simulink model "Simulink_asserv_Disc_15Mars"  (R2024a)
settings: Solver=VariableStepAuto  StartTime=0.0  StopTime=1000  FixedStep=0.01  RelTol=1e-3
model workspace (MAT data in the model file):
  AmbiantTemp = 25
  CondSig_mesureTemp_Gain = 4.35
  CondSig_mesureTemp_Vsub = 1.95
  DivTen_mesureTemp_R_pullup = 10000
  DivTen_mesureTemp_Vcc = 5
  Estimateur_alpha = 0.5
  Filtre_mesureTemp_deno = [0.0033 1]
  Gain_Comparateur_VoltageControle = 0.32
  RC_deno = [3.22e-08 3.04e-05 0.00955 1]
  SourceCourant_Gain_Vcontrole_vers_A = 3.1564
  ThermoRes_SHTEMP_A = 0.003354
  ThermoRes_SHTEMP_B = 0.00026
  ThermoRes_SHTEMP_C = 1.6e-06
  ThermoRes_SHTEMP_D = 6.3e-08
  ThermoRes_SH_A = -14.65719
  ThermoRes_SH_B = 4798.842
  ThermoRes_SH_C = -115334
  ThermoRes_SH_D = -3730535
  ThermoRes_SH_R_nom = 10000
  periodeEchant = 2
  setupDelay = 4
libraries: simulink x5
settings Model: SimulationMode=rapid-accelerator  Creator=alcot161  LastModifiedBy=ALCOT161

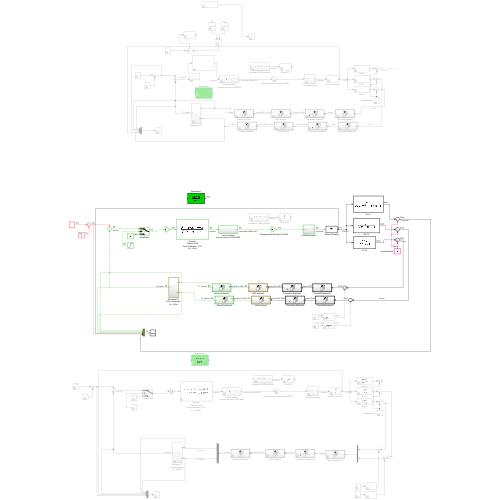
[thumbnail: Simulink's stored preview of the top-level diagram]
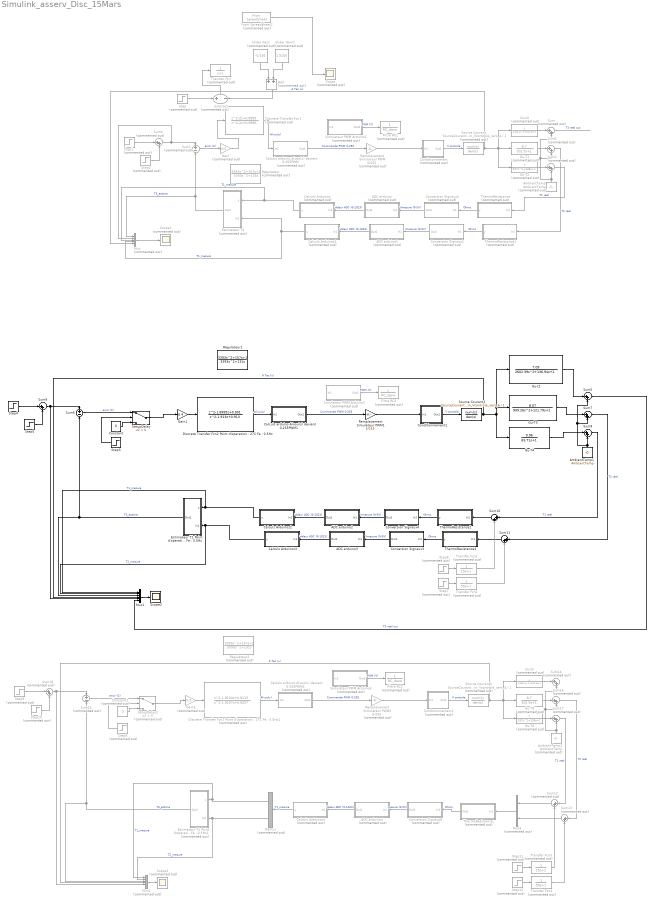
== system Simulink_asserv_Disc_15Mars ==
  ADC arduino : Subsystem  Commented=on  TreatAsAtomicUnit=on
  ADC arduino1 : Subsystem  Commented=on  TreatAsAtomicUnit=on
  ADC arduino2 : Subsystem  TreatAsAtomicUnit=on
  ADC arduino3 : Subsystem  TreatAsAtomicUnit=on
  ADC arduino4 : Subsystem  Commented=on  TreatAsAtomicUnit=on
  Add : Sum  Commented=on
  AmbiantTemp : Constant  Commented=on  Value=AmbiantTemp
  AmbiantTemp1 : Constant  Value=AmbiantTemp
  AmbiantTemp2 : Constant  Commented=on  Value=AmbiantTemp
  Calculs Arduinos : Subsystem  Commented=on  TreatAsAtomicUnit=on
  Calculs Arduinos1 : Subsystem  Commented=on  TreatAsAtomicUnit=on
  Calculs Arduinos2 : Subsystem  TreatAsAtomicUnit=on
  Calculs Arduinos3 : Subsystem  TreatAsAtomicUnit=on
  Calculs Arduinos4 : Subsystem  Commented=on  TreatAsAtomicUnit=on
  Calculs arduino A(voulu) devient 0-255PWM : Subsystem  Commented=on
  Calculs arduino A(voulu) devient 0-255PWM1 : Subsystem
  Calculs arduino A(voulu) devient 0-255PWM2 : Subsystem  Commented=on
  Conditionnement : Subsystem  Commented=on
  Conditionnement1 : Subsystem
  Conditionnement2 : Subsystem  Commented=on
  Constant : Constant  Value=0  SampleTime=periodeEchant
  Constant1 : Constant  Commented=on  Value=0  SampleTime=periodeEchant
  Conversion Signaux1 : Subsystem  Commented=on  TreatAsAtomicUnit=on
  Conversion Signaux2 : Subsystem  Commented=on  TreatAsAtomicUnit=on
  Conversion Signaux3 : Subsystem  TreatAsAtomicUnit=on
  Conversion Signaux4 : Subsystem  TreatAsAtomicUnit=on
  Conversion Signaux6 : Subsystem  Commented=on  TreatAsAtomicUnit=on
  Demux : Demux  Commented=on  Outputs=2
  Discrete Transfer Fcn1 : DiscreteTransferFcn  Commented=on  Numerator=[1 -2 0.9995]  Denominator=[1 -2 0.9996]
  "Discrete Transfer Fcn2 Point d'operation : 27C Fe : 0.5Hz" : DiscreteTransferFcn  Numerator=[1 -1.8995 0.901]  Denominator=[1 -1.913 0.913]
  "Discrete Transfer Fcn2 Point d'operation : 27C Fe : 0.5Hz1" : DiscreteTransferFcn  Commented=on  Numerator=[1 -1.9104 0.9115]  Denominator=[1 -1.9257 0.9257]
  "Estimateur T1 Point d'operation Fe : 0.5Hz" : Subsystem
  "Estimateur T1 Point d'operation Fe : 0.5Hz1" : Subsystem  Commented=on
  Estimateur T3 : Subsystem  Commented=on
  Filtre RC1 : TransferFcn  Commented=on  Denominator=RC_deno
  Filtre RC2 : TransferFcn  Commented=on  Denominator=RC_deno
  Filtre RC3 : TransferFcn  Commented=on  Denominator=RC_deno
  From Spreadsheet2 : FromSpreadsheet  Commented=on  FileName=N600_N800.xlsx  SheetName=P600_P800  Range=A2:A100  SampleTime=-1
  Gain : Gain  Commented=on  Gain=0.5
  Gain1 : Gain  Gain=0.4
  Gain2 : Gain  Commented=on  Gain=0.5
  Gu-T1 : TransferFcn  Commented=on  Numerator=[8.7]  Denominator=[102.5 1]
  Gu-T2 : TransferFcn  Commented=on  Numerator=[7]  Denominator=[537 138 1]
  Gu-T3 : TransferFcn  Numerator=[8.07]  Denominator=[909.26 121.79 1]
  Gu-T4 : TransferFcn  Numerator=[9.96]  Denominator=[83.71 1]
  Gu-T5 : TransferFcn  Commented=on  Numerator=[8.7]  Denominator=[102.5 1]
  Gu-T6 : TransferFcn  Commented=on  Numerator=[7]  Denominator=[537 138 1]
  Gu-t1 : TransferFcn  Numerator=[7.09]  Denominator=[2602.39 136.94 1]
  Gu-t2 : TransferFcn  Commented=on  Numerator=[6]  Denominator=[3403.4 156.9 1]
  Gu-t3 : TransferFcn  Commented=on  Numerator=[6]  Denominator=[3403.4 156.9 1]
  Mux : Mux  Commented=on  Inputs=5
  Mux1 : Mux  Inputs=6
  Mux2 : Mux  Commented=on  Inputs=6
  Mux3 : Mux  Commented=on  Inputs=2
  Remplacement Simulateur PWM : Gain  Commented=on  Gain=5/255
  Remplacement Simulateur PWM1 : Gain  Gain=5/255
  Remplacement Simulateur PWM2 : Gain  Commented=on  Gain=5/255
  Régulateur : TransferFcn  Commented=on  Numerator=[3393 157 1]  Denominator=[3393 131 0]
  Régulateur1 : TransferFcn  Numerator=[3393 157 1]  Denominator=[3393 131 0]
  Régulateur2 : TransferFcn  Commented=on  Numerator=[3393 157 1]  Denominator=[3393 131 0]
  Scope : Scope  Commented=on
  Scope1 : Scope  Commented=on
  Scope2 : Scope
  Scope3 : Scope  Commented=on
  SetupDelay : Switch  Criteria=u2 > Threshold  SaturateOnIntegerOverflow=off  InputSameDT=off
  SetupDelay1 : Switch  Commented=on  Criteria=u2 > Threshold  SaturateOnIntegerOverflow=off  InputSameDT=off
  Simulateur PWM Arduino1 : Subsystem  Commented=on
  Simulateur PWM Arduino2 : Subsystem  Commented=on
  Simulateur PWM Arduino3 : Subsystem  Commented=on
  Slider Gain : simulink/Math Operations/Slider Gain  Commented=on  gain=-0.516  low=-2  high=2
  Slider Gain1 : simulink/Math Operations/Slider Gain  Commented=on  gain=1.5155  low=-2  high=2
  Source Courant : TransferFcn  Commented=on  Numerator=SourceCourant_Gain_Vcontrole_vers_A  Denominator=1
  Source Courant1 : TransferFcn  Numerator=SourceCourant_Gain_Vcontrole_vers_A  Denominator=1
  Source Courant2 : TransferFcn  Commented=on  Numerator=SourceCourant_Gain_Vcontrole_vers_A  Denominator=1
  Step : Step  Commented=on  SampleTime=0
  Step1 : Step  Commented=on  Time=10  Before=25  After=27  SampleTime=0.05
  Step10 : Step  Commented=on  Time=500  After=-4  SampleTime=0.05
  Step11 : Step  Commented=on  Time=300  SampleTime=0
  Step12 : Step  Commented=on  Time=700  SampleTime=0
  Step2 : Step  Commented=on  Time=500  After=-4  SampleTime=0.05
  Step3 : Step  Time=setupDelay+1  SampleTime=periodeEchant
  Step4 : Step  Time=25  Before=25  After=27  SampleTime=0.05
  Step5 : Step  Time=500  After=-4  SampleTime=0.05
  Step6 : Step  Commented=on  Time=300  SampleTime=0
  Step7 : Step  Commented=on  Time=700  SampleTime=0
  Step8 : Step  Commented=on  Time=setupDelay+1  SampleTime=periodeEchant
  Step9 : Step  Commented=on  Time=25  Before=25  After=27  SampleTime=0.05
  Subtract : Sum  Commented=on  Inputs=+-
  Sum{,2..4,12..14,16..18} (10 alike) : Sum  Commented=on  Inputs=|++
  Sum1 : Sum  Commented=on  Inputs=+|-  SampleTime=0
  Sum{5,7..11} (6 alike) : Sum  Inputs=|++
  Sum15 : Sum  Commented=on  Inputs=+|-  SampleTime=2
  Sum6 : Sum  Inputs=+|-  SampleTime=2
  ThermoResistance : Subsystem  Commented=on  TreatAsAtomicUnit=on
  ThermoResistance1 : Subsystem  Commented=on  TreatAsAtomicUnit=on
  ThermoResistance2 : Subsystem  TreatAsAtomicUnit=on
  ThermoResistance3 : Subsystem  TreatAsAtomicUnit=on
  ThermoResistance_ : Subsystem  Commented=on  TreatAsAtomicUnit=on
  Transfer Fcn : TransferFcn  Commented=on  Denominator=[1 1]
  Transfer Fcn1 : TransferFcn  Commented=on  Denominator=[15 1]
  Transfer Fcn2 : TransferFcn  Commented=on  Denominator=[50 1]
  Transfer Fcn3 : TransferFcn  Commented=on  Denominator=[15 1]
  Transfer Fcn4 : TransferFcn  Commented=on  Denominator=[50 1]
  wires:
  From Spreadsheet2/1 -> Scope/1
  Subtract/1 -> Transfer Fcn/1
  Slider Gain/1 -> Add/1
  Slider Gain1/1 -> Add/2
  Add/1 -> Subtract/2
  Step/1 -> Subtract/1
  Sum1/1 -> Gain/1  "error (C)"
  Calculs arduino A(voulu) devient 0-255PWM/1(Out1) -> Remplacement Simulateur PWM/1  "Commande PWM 0-255"
  Remplacement Simulateur PWM/1 -> Conditionnement/1(In1)
  Conditionnement/1(Out1) -> Source Courant/1  "V controle"
  Source Courant/1 -> Mux/5, Gu-T2/1, Gu-T1/1, Gu-t3/1  "A Tec (u)"
  Gu-t3/1 -> Sum/1
  Gu-T1/1 -> Sum2/1
  Gu-T2/1 -> Sum3/1
  AmbiantTemp/1 -> Sum/2, Sum2/2, Sum3/2
  Sum2/1 -> ThermoResistance1/1(In1)  "T2 reel"
  Sum3/1 -> ThermoResistance/1(In1)  "T1 reel"
  ThermoResistance/1(y) -> Conversion Signaux2/1(In1)  "Ohms"
  Conversion Signaux2/1(Out1) -> ADC arduino/1(In1)  "Vmesure (0-5V)"
  ADC arduino/1(Out1) -> Calculs Arduinos/1(In1)  "Valeur ADC (0-1023)"
  Calculs Arduinos/1(y) -> Mux/3, Estimateur T3/1(y)  "T1_mesure"
  Estimateur T3/1(Out1) -> Mux/1, Sum1/2  "T3_estime"
  Simulateur PWM Arduino1/1(Out1) -> Filtre RC1/1  "PWM (V)"
  Sum/1 -> ?  "T3 reel out"
  Gain/1 -> Discrete Transfer Fcn1/1
  Discrete Transfer Fcn1/1 -> Calculs arduino A(voulu) devient 0-255PWM/1(In1)  "A(voulu)"
  Step1/1 -> Sum4/1
  Step2/1 -> Sum4/2
  Mux/1 -> Scope1/1
  Sum4/1 -> Mux/2, Sum1/1
  Calculs Arduinos1/1(y) -> Estimateur T3/2(In2), Mux/4  "T1_mesure"
  ThermoResistance1/1(y) -> Conversion Signaux1/1(In1)  "Ohms"
  ADC arduino1/1(Out1) -> Calculs Arduinos1/1(In1)  "Valeur ADC (0-1023)"
  Conversion Signaux1/1(Out1) -> ADC arduino1/1(In1)  "Vmesure (0-5V)"
  ThermoResistance3/1(y) -> Conversion Signaux3/1(In1)  "Ohms"
  Step4/1 -> Sum9/1
  Gu-T3/1 -> Sum7/1
  Conversion Signaux3/1(Out1) -> ADC arduino3/1(In1)  "Vmesure (0-5V)"
  Sum9/1 -> Sum6/1, Mux1/5
  ADC arduino3/1(Out1) -> Calculs Arduinos3/1(In1)  "Valeur ADC (0-1023)"
  Simulateur PWM Arduino2/1(Out1) -> Filtre RC2/1  "PWM (V)"
  Step5/1 -> Sum9/2
  Conversion Signaux4/1(Out1) -> ADC arduino2/1(In1)  "Vmesure (0-5V)"
  AmbiantTemp1/1 -> Sum5/2, Sum7/2, Sum8/2
  Remplacement Simulateur PWM1/1 -> Conditionnement1/1(In1)
  Calculs Arduinos2/1(y) -> Mux1/1, "Estimateur T1 Point d'operation Fe : 0.5Hz"/1(y)  "T1_mesure"
  ADC arduino2/1(Out1) -> Calculs Arduinos2/1(In1)  "Valeur ADC (0-1023)"
  Calculs arduino A(voulu) devient 0-255PWM1/1(Out1) -> Remplacement Simulateur PWM1/1  "Commande PWM 0-255"
  Calculs Arduinos3/1(y) -> Mux1/2, "Estimateur T1 Point d'operation Fe : 0.5Hz"/2(In2)  "T2_mesure"
  Source Courant1/1 -> Mux1/4, Gu-T3/1, Gu-t1/1, Gu-T4/1  "A Tec (u)"
  ThermoResistance2/1(y) -> Conversion Signaux4/1(In1)  "Ohms"
  Sum7/1 -> Sum11/1  "T2 reel"
  Conditionnement1/1(Out1) -> Source Courant1/1  "V controle"
  Gu-T4/1 -> Sum8/1
  Gu-t1/1 -> Sum5/1
  "Discrete Transfer Fcn2 Point d'operation : 27C Fe : 0.5Hz"/1 -> Calculs arduino A(voulu) devient 0-255PWM1/1(In1)  "A(voulu)"
  "Estimateur T1 Point d'operation Fe : 0.5Hz"/1(Out1) -> Mux1/3, Sum6/2  "T3_estime"
  Mux1/1 -> Scope2/1
  Step3/1 -> SetupDelay/2
  Gain1/1 -> "Discrete Transfer Fcn2 Point d'operation : 27C Fe : 0.5Hz"/1
  Sum6/1 -> SetupDelay/1  "error (C)"
  SetupDelay/1 -> Gain1/1
  Constant/1 -> SetupDelay/3
  Sum8/1 -> Sum10/1  "T1 reel"
  Step6/1 -> Transfer Fcn1/1
  Sum10/1 -> ThermoResistance2/1(In1)
  Sum11/1 -> ThermoResistance3/1(In1)
  Step7/1 -> Transfer Fcn2/1
  Transfer Fcn1/1 -> Sum10/2
  Transfer Fcn2/1 -> Sum11/2
  Transfer Fcn3/1 -> Sum12/2
  Step8/1 -> SetupDelay1/2
  Step9/1 -> Sum18/1
  Sum18/1 -> Sum15/1, Mux2/5
  Source Courant2/1 -> Mux2/4, Gu-T6/1, Gu-T5/1, Gu-t2/1  "A Tec (u)"
  Constant1/1 -> SetupDelay1/3
  Step10/1 -> Sum18/2
  Conditionnement2/1(Out1) -> Source Courant2/1  "V controle"
  Mux2/1 -> Scope3/1
  Demux/1 -> Mux2/1, "Estimateur T1 Point d'operation Fe : 0.5Hz1"/1(y)  "T1_mesure"
  "Discrete Transfer Fcn2 Point d'operation : 27C Fe : 0.5Hz1"/1 -> Calculs arduino A(voulu) devient 0-255PWM2/1(In1)  "A(voulu)"
  Simulateur PWM Arduino3/1(Out1) -> Filtre RC3/1  "PWM (V)"
  Gu-T6/1 -> Sum17/1
  Sum17/1 -> Sum12/1  "T1 reel"
  Remplacement Simulateur PWM2/1 -> Conditionnement2/1(In1)
  "Estimateur T1 Point d'operation Fe : 0.5Hz1"/1(Out1) -> Mux2/3, Sum15/2  "T3_estime"
  Calculs arduino A(voulu) devient 0-255PWM2/1(Out1) -> Remplacement Simulateur PWM2/1  "Commande PWM 0-255"
  ThermoResistance_/1(Out1) -> Conversion Signaux6/1(In1)  "Ohms"
  Demux/2 -> Mux2/2, "Estimateur T1 Point d'operation Fe : 0.5Hz1"/2(In2)  "T2_mesure"
  Sum15/1 -> SetupDelay1/1  "error (C)"
  SetupDelay1/1 -> Gain2/1
  Step12/1 -> Transfer Fcn4/1
  Gu-T5/1 -> Sum16/1
  Step11/1 -> Transfer Fcn3/1
  Gain2/1 -> "Discrete Transfer Fcn2 Point d'operation : 27C Fe : 0.5Hz1"/1
  AmbiantTemp2/1 -> Sum14/2, Sum16/2, Sum17/2
  Sum12/1 -> Mux3/1
  Sum13/1 -> Mux3/2
  Sum16/1 -> Sum13/1  "T2 reel"
  Transfer Fcn4/1 -> Sum13/2
  Gu-t2/1 -> Sum14/1
  Mux3/1 -> ThermoResistance_/1(In1)
  Calculs Arduinos4/1(y) -> Demux/1  "T1_mesure"
  ADC arduino4/1(Out1) -> Calculs Arduinos4/1(In1)  "Valeur ADC (0-1023)"
  Conversion Signaux6/1(Out1) -> ADC arduino4/1(In1)  "mesure (0-5V)"
  Sum5/1 -> Mux1/6  "T3 reel out"

== system Simulink_asserv_Disc_15Mars/ADC arduino ==
  In1 : Inport  Partition=on  PartitionDimension=1  PartitionWidth=1  PartitionOffset=0
  Floor : Rounding
  For Each : ForEach  DisableCoverage=on
  Gain : Gain  Gain=1024/5
  Out1 : Outport  ConcatenationDimension=1
  wires:
  In1/1 -> Gain/1
  Gain/1 -> Floor/1
  Floor/1 -> Out1/1

== system Simulink_asserv_Disc_15Mars/ADC arduino1 ==
  In1 : Inport  Partition=on  PartitionDimension=1  PartitionWidth=1  PartitionOffset=0
  Floor : Rounding
  For Each : ForEach  DisableCoverage=on
  Gain : Gain  Gain=1024/5
  Out1 : Outport  ConcatenationDimension=1
  wires:
  In1/1 -> Gain/1
  Gain/1 -> Floor/1
  Floor/1 -> Out1/1

== system Simulink_asserv_Disc_15Mars/ADC arduino2 ==
  In1 : Inport  Partition=on  PartitionDimension=1  PartitionWidth=1  PartitionOffset=0
  Floor : Rounding
  For Each : ForEach  DisableCoverage=on
  Gain : Gain  Gain=1024/5
  Setup fonction delay : Step  Time=setupDelay-2  SampleTime=0
  Switch : Switch  Criteria=u2 > Threshold  SaturateOnIntegerOverflow=off  InputSameDT=off
  Out1 : Outport  SampleTime=periodeEchant  ConcatenationDimension=1
  wires:
  In1/1 -> Gain/1
  Gain/1 -> Floor/1
  Floor/1 -> Out1/1
  Setup fonction delay/1 -> Switch/2

== system Simulink_asserv_Disc_15Mars/ADC arduino3 ==
  In1 : Inport  Partition=on  PartitionDimension=1  PartitionWidth=1  PartitionOffset=0
  Floor : Rounding
  For Each : ForEach  DisableCoverage=on
  Gain : Gain  Gain=1024/5
  Setup fonction delay : Step  Time=setupDelay-2  SampleTime=0
  Switch : Switch  Criteria=u2 > Threshold  SaturateOnIntegerOverflow=off  InputSameDT=off
  Out1 : Outport  SampleTime=periodeEchant  ConcatenationDimension=1
  wires:
  In1/1 -> Gain/1
  Gain/1 -> Floor/1
  Floor/1 -> Out1/1
  Setup fonction delay/1 -> Switch/2

== system Simulink_asserv_Disc_15Mars/ADC arduino4 ==
  In1 : Inport  Partition=on  PartitionDimension=1  PartitionWidth=1  PartitionOffset=0
  Floor : Rounding
  For Each : ForEach  DisableCoverage=on
  Gain : Gain  Gain=1024/5
  Out1 : Outport  SampleTime=periodeEchant  ConcatenationDimension=1
  wires:
  In1/1 -> Gain/1
  Gain/1 -> Floor/1
  Floor/1 -> Out1/1

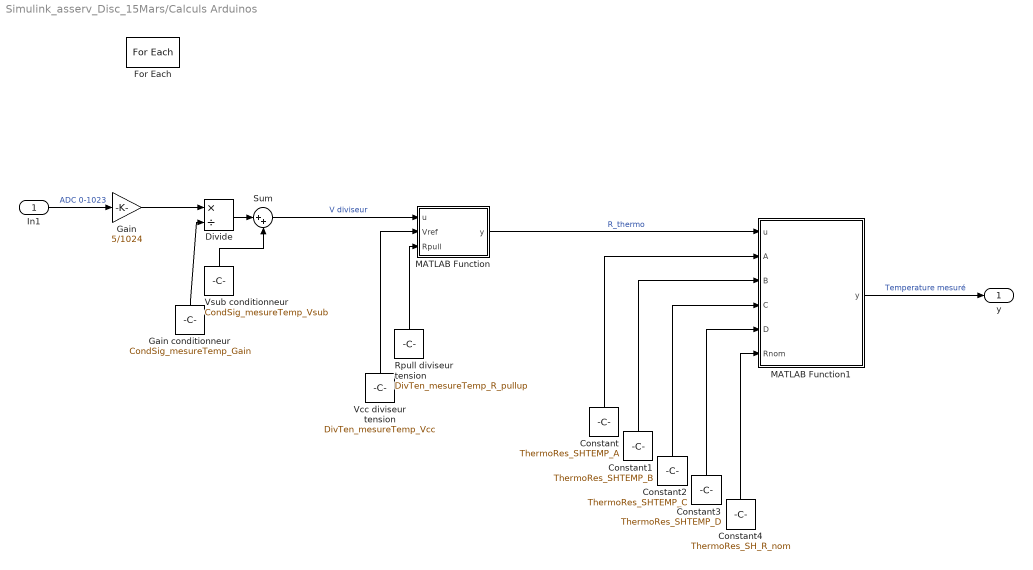
== system Simulink_asserv_Disc_15Mars/Calculs Arduinos ==
  In1 : Inport  Partition=on  PartitionDimension=1  PartitionWidth=1  PartitionOffset=0
  Constant : Constant  Value=ThermoRes_SHTEMP_A
  Constant1 : Constant  Value=ThermoRes_SHTEMP_B
  Constant2 : Constant  Value=ThermoRes_SHTEMP_C
  Constant3 : Constant  Value=ThermoRes_SHTEMP_D
  Constant4 : Constant  Value=ThermoRes_SH_R_nom
  Divide : Product  Inputs=*/
  For Each : ForEach  DisableCoverage=on
  Gain : Gain  Gain=5/1024
  Gain conditionneur : Constant  Value=CondSig_mesureTemp_Gain
  MATLAB Function : MATLAB Function  TreatAsAtomicUnit=on
  MATLAB Function1 : MATLAB Function  TreatAsAtomicUnit=on
  Rpull diviseur tension : Constant  Value=DivTen_mesureTemp_R_pullup
  Sum : Sum  Inputs=|++
  Vcc diviseur tension : Constant  Value=DivTen_mesureTemp_Vcc
  Vsub conditionneur : Constant  Value=CondSig_mesureTemp_Vsub
  y : Outport  ConcatenationDimension=1
  wires:
  In1/1 -> Gain/1  "ADC 0-1023"
  Gain/1 -> Divide/1
  Gain conditionneur/1 -> Divide/2
  Divide/1 -> Sum/1
  Vsub conditionneur/1 -> Sum/2
  Sum/1 -> MATLAB Function/1(u)  "V diviseur"
  Rpull diviseur tension/1 -> MATLAB Function/3(Rpull)
  Vcc diviseur tension/1 -> MATLAB Function/2(Vref)
  MATLAB Function/1(y) -> MATLAB Function1/1(u)  "R_thermo"
  Constant/1 -> MATLAB Function1/2(A)
  Constant1/1 -> MATLAB Function1/3(B)
  Constant2/1 -> MATLAB Function1/4(C)
  Constant3/1 -> MATLAB Function1/5(D)
  Constant4/1 -> MATLAB Function1/6(Rnom)
  MATLAB Function1/1(y) -> y/1  "Temperature mesuré"

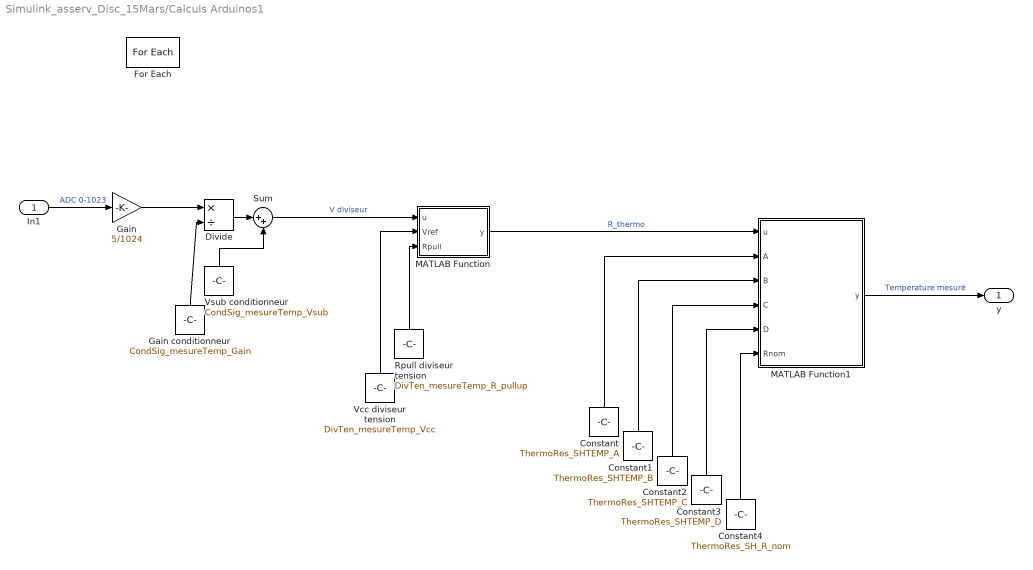
== system Simulink_asserv_Disc_15Mars/Calculs Arduinos1 ==
  In1 : Inport  Partition=on  PartitionDimension=1  PartitionWidth=1  PartitionOffset=0
  Constant : Constant  Value=ThermoRes_SHTEMP_A
  Constant1 : Constant  Value=ThermoRes_SHTEMP_B
  Constant2 : Constant  Value=ThermoRes_SHTEMP_C
  Constant3 : Constant  Value=ThermoRes_SHTEMP_D
  Constant4 : Constant  Value=ThermoRes_SH_R_nom
  Divide : Product  Inputs=*/
  For Each : ForEach  DisableCoverage=on
  Gain : Gain  Gain=5/1024
  Gain conditionneur : Constant  Value=CondSig_mesureTemp_Gain
  MATLAB Function : MATLAB Function  TreatAsAtomicUnit=on
  MATLAB Function1 : MATLAB Function  TreatAsAtomicUnit=on
  Rpull diviseur tension : Constant  Value=DivTen_mesureTemp_R_pullup
  Sum : Sum  Inputs=|++
  Vcc diviseur tension : Constant  Value=DivTen_mesureTemp_Vcc
  Vsub conditionneur : Constant  Value=CondSig_mesureTemp_Vsub
  y : Outport  ConcatenationDimension=1
  wires:
  In1/1 -> Gain/1  "ADC 0-1023"
  Gain/1 -> Divide/1
  Gain conditionneur/1 -> Divide/2
  Divide/1 -> Sum/1
  Vsub conditionneur/1 -> Sum/2
  Sum/1 -> MATLAB Function/1(u)  "V diviseur"
  Rpull diviseur tension/1 -> MATLAB Function/3(Rpull)
  Vcc diviseur tension/1 -> MATLAB Function/2(Vref)
  MATLAB Function/1(y) -> MATLAB Function1/1(u)  "R_thermo"
  Constant/1 -> MATLAB Function1/2(A)
  Constant1/1 -> MATLAB Function1/3(B)
  Constant2/1 -> MATLAB Function1/4(C)
  Constant3/1 -> MATLAB Function1/5(D)
  Constant4/1 -> MATLAB Function1/6(Rnom)
  MATLAB Function1/1(y) -> y/1  "Temperature mesuré"

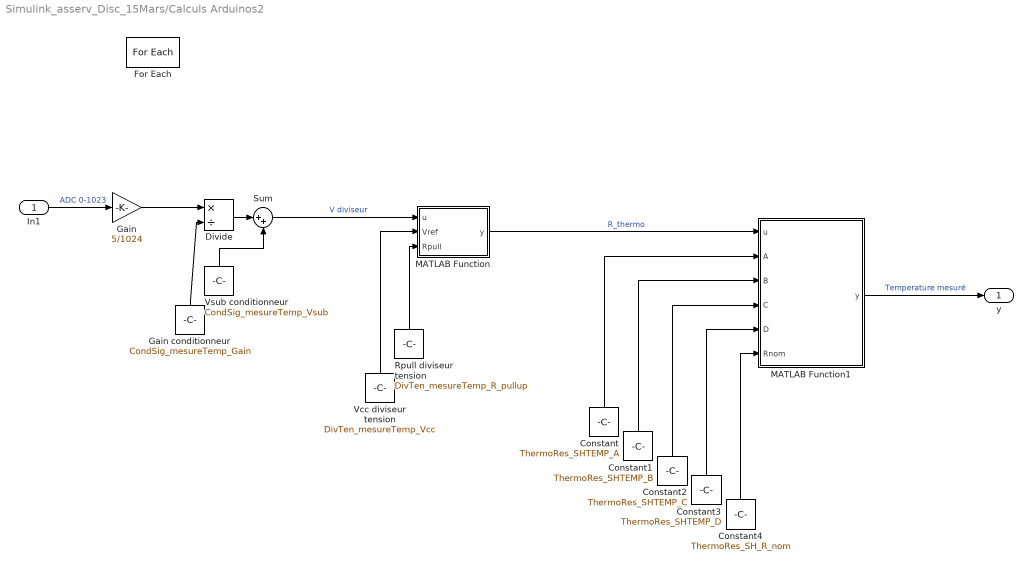
== system Simulink_asserv_Disc_15Mars/Calculs Arduinos2 ==
  In1 : Inport  Partition=on  PartitionDimension=1  PartitionWidth=1  PartitionOffset=0
  Constant : Constant  Value=ThermoRes_SHTEMP_A
  Constant1 : Constant  Value=ThermoRes_SHTEMP_B
  Constant2 : Constant  Value=ThermoRes_SHTEMP_C
  Constant3 : Constant  Value=ThermoRes_SHTEMP_D
  Constant4 : Constant  Value=ThermoRes_SH_R_nom
  Divide : Product  Inputs=*/
  For Each : ForEach  DisableCoverage=on
  Gain : Gain  Gain=5/1024
  Gain conditionneur : Constant  Value=CondSig_mesureTemp_Gain
  MATLAB Function : MATLAB Function  TreatAsAtomicUnit=on
  MATLAB Function1 : MATLAB Function  TreatAsAtomicUnit=on
  Rpull diviseur tension : Constant  Value=DivTen_mesureTemp_R_pullup
  Sum : Sum  Inputs=|++
  Vcc diviseur tension : Constant  Value=DivTen_mesureTemp_Vcc
  Vsub conditionneur : Constant  Value=CondSig_mesureTemp_Vsub
  y : Outport  ConcatenationDimension=1
  wires:
  In1/1 -> Gain/1  "ADC 0-1023"
  Gain/1 -> Divide/1
  Gain conditionneur/1 -> Divide/2
  Divide/1 -> Sum/1
  Vsub conditionneur/1 -> Sum/2
  Sum/1 -> MATLAB Function/1(u)  "V diviseur"
  Rpull diviseur tension/1 -> MATLAB Function/3(Rpull)
  Vcc diviseur tension/1 -> MATLAB Function/2(Vref)
  MATLAB Function/1(y) -> MATLAB Function1/1(u)  "R_thermo"
  Constant/1 -> MATLAB Function1/2(A)
  Constant1/1 -> MATLAB Function1/3(B)
  Constant2/1 -> MATLAB Function1/4(C)
  Constant3/1 -> MATLAB Function1/5(D)
  Constant4/1 -> MATLAB Function1/6(Rnom)
  MATLAB Function1/1(y) -> y/1  "Temperature mesuré"

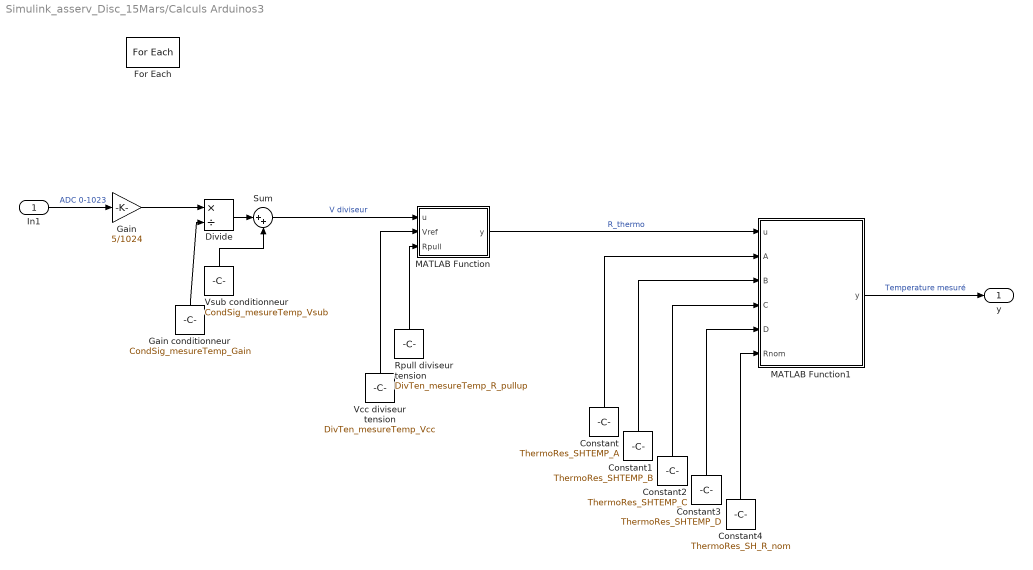
== system Simulink_asserv_Disc_15Mars/Calculs Arduinos3 ==
  In1 : Inport  Partition=on  PartitionDimension=1  PartitionWidth=1  PartitionOffset=0
  Constant : Constant  Value=ThermoRes_SHTEMP_A
  Constant1 : Constant  Value=ThermoRes_SHTEMP_B
  Constant2 : Constant  Value=ThermoRes_SHTEMP_C
  Constant3 : Constant  Value=ThermoRes_SHTEMP_D
  Constant4 : Constant  Value=ThermoRes_SH_R_nom
  Divide : Product  Inputs=*/
  For Each : ForEach  DisableCoverage=on
  Gain : Gain  Gain=5/1024
  Gain conditionneur : Constant  Value=CondSig_mesureTemp_Gain
  MATLAB Function : MATLAB Function  TreatAsAtomicUnit=on
  MATLAB Function1 : MATLAB Function  TreatAsAtomicUnit=on
  Rpull diviseur tension : Constant  Value=DivTen_mesureTemp_R_pullup
  Sum : Sum  Inputs=|++
  Vcc diviseur tension : Constant  Value=DivTen_mesureTemp_Vcc
  Vsub conditionneur : Constant  Value=CondSig_mesureTemp_Vsub
  y : Outport  ConcatenationDimension=1
  wires:
  In1/1 -> Gain/1  "ADC 0-1023"
  Gain/1 -> Divide/1
  Gain conditionneur/1 -> Divide/2
  Divide/1 -> Sum/1
  Vsub conditionneur/1 -> Sum/2
  Sum/1 -> MATLAB Function/1(u)  "V diviseur"
  Rpull diviseur tension/1 -> MATLAB Function/3(Rpull)
  Vcc diviseur tension/1 -> MATLAB Function/2(Vref)
  MATLAB Function/1(y) -> MATLAB Function1/1(u)  "R_thermo"
  Constant/1 -> MATLAB Function1/2(A)
  Constant1/1 -> MATLAB Function1/3(B)
  Constant2/1 -> MATLAB Function1/4(C)
  Constant3/1 -> MATLAB Function1/5(D)
  Constant4/1 -> MATLAB Function1/6(Rnom)
  MATLAB Function1/1(y) -> y/1  "Temperature mesuré"

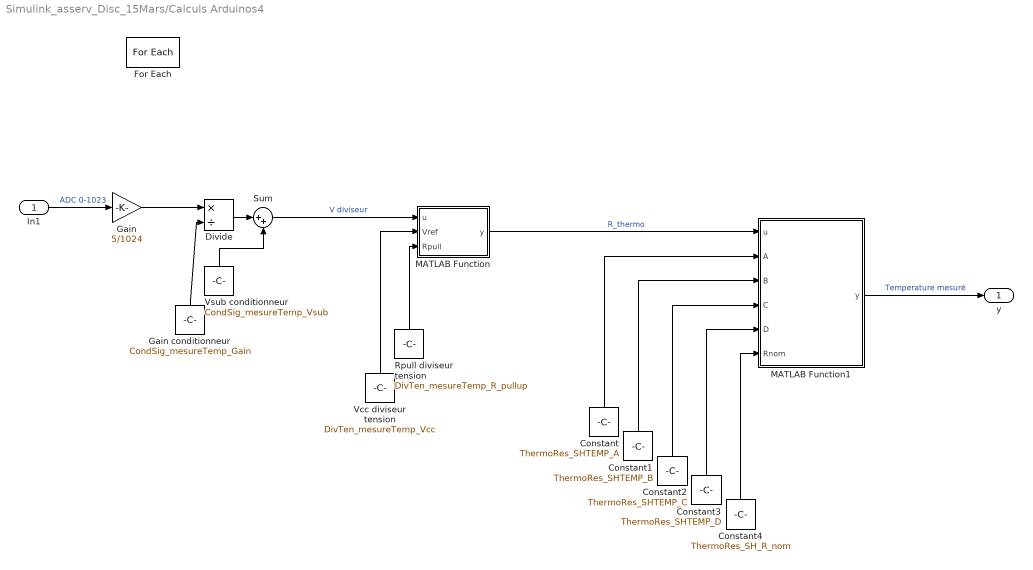
== system Simulink_asserv_Disc_15Mars/Calculs Arduinos4 ==
  In1 : Inport  Partition=on  PartitionDimension=1  PartitionWidth=1  PartitionOffset=0
  Constant : Constant  Value=ThermoRes_SHTEMP_A
  Constant1 : Constant  Value=ThermoRes_SHTEMP_B
  Constant2 : Constant  Value=ThermoRes_SHTEMP_C
  Constant3 : Constant  Value=ThermoRes_SHTEMP_D
  Constant4 : Constant  Value=ThermoRes_SH_R_nom
  Divide : Product  Inputs=*/
  For Each : ForEach  DisableCoverage=on
  Gain : Gain  Gain=5/1024
  Gain conditionneur : Constant  Value=CondSig_mesureTemp_Gain
  MATLAB Function : MATLAB Function  TreatAsAtomicUnit=on
  MATLAB Function1 : MATLAB Function  TreatAsAtomicUnit=on
  Rpull diviseur tension : Constant  Value=DivTen_mesureTemp_R_pullup
  Sum : Sum  Inputs=|++
  Vcc diviseur tension : Constant  Value=DivTen_mesureTemp_Vcc
  Vsub conditionneur : Constant  Value=CondSig_mesureTemp_Vsub
  y : Outport  ConcatenationDimension=1
  wires:
  In1/1 -> Gain/1  "ADC 0-1023"
  Gain/1 -> Divide/1
  Gain conditionneur/1 -> Divide/2
  Divide/1 -> Sum/1
  Vsub conditionneur/1 -> Sum/2
  Sum/1 -> MATLAB Function/1(u)  "V diviseur"
  Rpull diviseur tension/1 -> MATLAB Function/3(Rpull)
  Vcc diviseur tension/1 -> MATLAB Function/2(Vref)
  MATLAB Function/1(y) -> MATLAB Function1/1(u)  "R_thermo"
  Constant/1 -> MATLAB Function1/2(A)
  Constant1/1 -> MATLAB Function1/3(B)
  Constant2/1 -> MATLAB Function1/4(C)
  Constant3/1 -> MATLAB Function1/5(D)
  Constant4/1 -> MATLAB Function1/6(Rnom)
  MATLAB Function1/1(y) -> y/1  "Temperature mesuré"

== system Simulink_asserv_Disc_15Mars/Calculs arduino A(voulu) devient 0-255PWM ==
  In1 : Inport
  Constante de centre : Constant  Value=0.8323
  Gain : Gain  Gain=0.3168166265365
  Gain1 : Gain  Gain=59.88
  Gain2 : Gain  Gain=2.56  ParamMin=0  ParamMax=255.9  OutMin=[0]  OutMax=[255]
  Rounding Function : Rounding
  Saturation : Saturate  UpperLimit=255  LowerLimit=0  LinearizeAsGain=off
  Sum : Sum  Inputs=|++
  Out1 : Outport
  wires:
  In1/1 -> Gain/1  "A_voulu"
  Gain/1 -> Sum/1  "V_controle_voulu -0.8V - 0.8V"
  Sum/1 -> Gain1/1
  Constante de centre/1 -> Sum/2
  Gain1/1 -> Gain2/1  "DutyCycle%"
  Gain2/1 -> Rounding Function/1
  Rounding Function/1 -> Saturation/1
  Saturation/1 -> Out1/1  "0-255"

== system Simulink_asserv_Disc_15Mars/Calculs arduino A(voulu) devient 0-255PWM1 ==
  In1 : Inport
  Constante de centre : Constant  Value=0.8323
  Gain : Gain  Gain=0.3168166265365
  Gain1 : Gain  Gain=59.88
  Gain2 : Gain  Gain=2.56  ParamMin=0  ParamMax=255.9  OutMin=[0]  OutMax=[255]
  Rounding Function : Rounding
  Saturation : Saturate  UpperLimit=255  LowerLimit=0  LinearizeAsGain=off
  Sum : Sum  Inputs=|++
  Out1 : Outport
  wires:
  In1/1 -> Gain/1  "A_voulu"
  Gain/1 -> Sum/1  "V_controle_voulu -0.8V - 0.8V"
  Sum/1 -> Gain1/1
  Constante de centre/1 -> Sum/2
  Gain1/1 -> Gain2/1  "DutyCycle%"
  Gain2/1 -> Rounding Function/1
  Rounding Function/1 -> Saturation/1
  Saturation/1 -> Out1/1  "0-255"

== system Simulink_asserv_Disc_15Mars/Calculs arduino A(voulu) devient 0-255PWM2 ==
  In1 : Inport
  Constante de centre : Constant  Value=0.8323
  Gain : Gain  Gain=0.3168166265365
  Gain1 : Gain  Gain=59.88
  Gain2 : Gain  Gain=2.56  ParamMin=0  ParamMax=255.9  OutMin=[0]  OutMax=[255]
  Rounding Function : Rounding
  Saturation : Saturate  UpperLimit=255  LowerLimit=0  LinearizeAsGain=off
  Sum : Sum  Inputs=|++
  Out1 : Outport
  wires:
  In1/1 -> Gain/1  "A_voulu"
  Gain/1 -> Sum/1  "V_controle_voulu -0.8V - 0.8V"
  Sum/1 -> Gain1/1
  Constante de centre/1 -> Sum/2
  Gain1/1 -> Gain2/1  "DutyCycle%"
  Gain2/1 -> Rounding Function/1
  Rounding Function/1 -> Saturation/1
  Saturation/1 -> Out1/1  "0-255"

== system Simulink_asserv_Disc_15Mars/Conditionnement ==
  In1 : Inport
  Constant : Constant  Value=2.5
  Gain : Gain  Gain=Gain_Comparateur_VoltageControle
  Subtract : Sum  Inputs=+-
  Out1 : Outport
  wires:
  In1/1 -> Subtract/1
  Constant/1 -> Subtract/2
  Subtract/1 -> Gain/1
  Gain/1 -> Out1/1

== system Simulink_asserv_Disc_15Mars/Conditionnement1 ==
  In1 : Inport
  Constant : Constant  Value=2.5
  Gain : Gain  Gain=Gain_Comparateur_VoltageControle
  Subtract : Sum  Inputs=+-
  Out1 : Outport
  wires:
  In1/1 -> Subtract/1
  Constant/1 -> Subtract/2
  Subtract/1 -> Gain/1
  Gain/1 -> Out1/1

== system Simulink_asserv_Disc_15Mars/Conditionnement2 ==
  In1 : Inport
  Constant : Constant  Value=2.5
  Gain : Gain  Gain=Gain_Comparateur_VoltageControle
  Subtract : Sum  Inputs=+-
  Out1 : Outport
  wires:
  In1/1 -> Subtract/1
  Constant/1 -> Subtract/2
  Subtract/1 -> Gain/1
  Gain/1 -> Out1/1

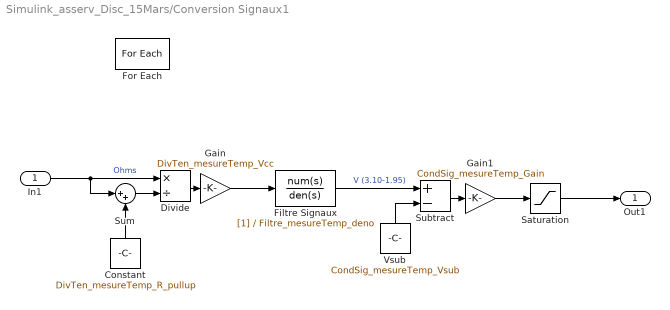
== system Simulink_asserv_Disc_15Mars/Conversion Signaux1 ==
  In1 : Inport  Partition=on  PartitionDimension=1  PartitionWidth=1  PartitionOffset=0
  Constant : Constant  Value=DivTen_mesureTemp_R_pullup
  Divide : Product  Inputs=*/
  Filtre Signaux : TransferFcn  Denominator=Filtre_mesureTemp_deno
  For Each : ForEach  DisableCoverage=on
  Gain : Gain  Gain=DivTen_mesureTemp_Vcc
  Gain1 : Gain  Gain=CondSig_mesureTemp_Gain
  Saturation : Saturate  UpperLimit=5  LowerLimit=0
  Subtract : Sum  Inputs=+-
  Sum : Sum  Inputs=|++
  Vsub : Constant  Value=CondSig_mesureTemp_Vsub
  Out1 : Outport  ConcatenationDimension=1
  wires:
  In1/1 -> Sum/1, Divide/1  "Ohms"
  Sum/1 -> Divide/2
  Constant/1 -> Sum/2
  Divide/1 -> Gain/1
  Gain/1 -> Filtre Signaux/1
  Vsub/1 -> Subtract/2
  Filtre Signaux/1 -> Subtract/1  "V (3.10-1.95)"
  Subtract/1 -> Gain1/1
  Gain1/1 -> Saturation/1
  Saturation/1 -> Out1/1

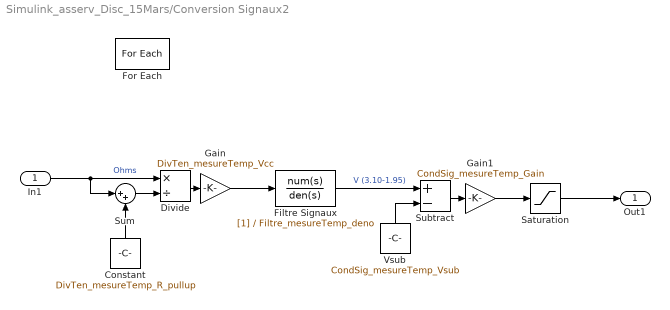
== system Simulink_asserv_Disc_15Mars/Conversion Signaux2 ==
  In1 : Inport  Partition=on  PartitionDimension=1  PartitionWidth=1  PartitionOffset=0
  Constant : Constant  Value=DivTen_mesureTemp_R_pullup
  Divide : Product  Inputs=*/
  Filtre Signaux : TransferFcn  Denominator=Filtre_mesureTemp_deno
  For Each : ForEach  DisableCoverage=on
  Gain : Gain  Gain=DivTen_mesureTemp_Vcc
  Gain1 : Gain  Gain=CondSig_mesureTemp_Gain
  Saturation : Saturate  UpperLimit=5  LowerLimit=0
  Subtract : Sum  Inputs=+-
  Sum : Sum  Inputs=|++
  Vsub : Constant  Value=CondSig_mesureTemp_Vsub
  Out1 : Outport  ConcatenationDimension=1
  wires:
  In1/1 -> Sum/1, Divide/1  "Ohms"
  Sum/1 -> Divide/2
  Constant/1 -> Sum/2
  Divide/1 -> Gain/1
  Gain/1 -> Filtre Signaux/1
  Vsub/1 -> Subtract/2
  Filtre Signaux/1 -> Subtract/1  "V (3.10-1.95)"
  Subtract/1 -> Gain1/1
  Gain1/1 -> Saturation/1
  Saturation/1 -> Out1/1

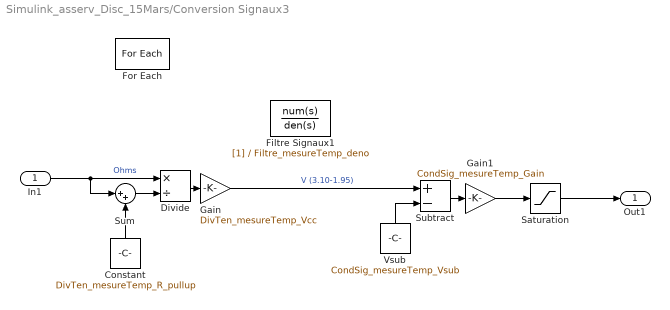
== system Simulink_asserv_Disc_15Mars/Conversion Signaux3 ==
  In1 : Inport  Partition=on  PartitionDimension=1  PartitionWidth=1  PartitionOffset=0
  Constant : Constant  Value=DivTen_mesureTemp_R_pullup
  Divide : Product  Inputs=*/
  Filtre Signaux1 : TransferFcn  Denominator=Filtre_mesureTemp_deno
  For Each : ForEach  DisableCoverage=on
  Gain : Gain  Gain=DivTen_mesureTemp_Vcc
  Gain1 : Gain  Gain=CondSig_mesureTemp_Gain
  Saturation : Saturate  UpperLimit=5  LowerLimit=0
  Subtract : Sum  Inputs=+-
  Sum : Sum  Inputs=|++
  Vsub : Constant  Value=CondSig_mesureTemp_Vsub
  Out1 : Outport  ConcatenationDimension=1
  wires:
  In1/1 -> Sum/1, Divide/1  "Ohms"
  Sum/1 -> Divide/2
  Constant/1 -> Sum/2
  Divide/1 -> Gain/1
  Vsub/1 -> Subtract/2
  Subtract/1 -> Gain1/1
  Gain1/1 -> Saturation/1
  Saturation/1 -> Out1/1
  Gain/1 -> Subtract/1  "V (3.10-1.95)"

== system Simulink_asserv_Disc_15Mars/Conversion Signaux4 ==
  In1 : Inport  Partition=on  PartitionDimension=1  PartitionWidth=1  PartitionOffset=0
  Constant : Constant  Value=DivTen_mesureTemp_R_pullup
  Divide : Product  Inputs=*/
  Filtre Signaux1 : TransferFcn  Denominator=Filtre_mesureTemp_deno
  For Each : ForEach  DisableCoverage=on
  Gain : Gain  Gain=DivTen_mesureTemp_Vcc
  Gain1 : Gain  Gain=CondSig_mesureTemp_Gain
  Saturation : Saturate  UpperLimit=5  LowerLimit=0
  Subtract : Sum  Inputs=+-
  Sum : Sum  Inputs=|++
  Vsub : Constant  Value=CondSig_mesureTemp_Vsub
  Out1 : Outport  ConcatenationDimension=1
  wires:
  In1/1 -> Sum/1, Divide/1  "Ohms"
  Sum/1 -> Divide/2
  Constant/1 -> Sum/2
  Divide/1 -> Gain/1
  Vsub/1 -> Subtract/2
  Subtract/1 -> Gain1/1
  Gain1/1 -> Saturation/1
  Saturation/1 -> Out1/1
  Gain/1 -> Subtract/1  "V (3.10-1.95)"

== system Simulink_asserv_Disc_15Mars/Conversion Signaux6 ==
  In1 : Inport  Partition=on  PartitionDimension=1  PartitionWidth=1  PartitionOffset=0
  Constant : Constant  Value=DivTen_mesureTemp_R_pullup
  Divide : Product  Inputs=*/
  Filtre Signaux1 : TransferFcn  Denominator=Filtre_mesureTemp_deno
  For Each : ForEach  DisableCoverage=on
  Gain : Gain  Gain=DivTen_mesureTemp_Vcc
  Gain1 : Gain  Gain=CondSig_mesureTemp_Gain
  Saturation : Saturate  UpperLimit=5  LowerLimit=0
  Subtract : Sum  Inputs=+-
  Sum : Sum  Inputs=|++
  Vsub : Constant  Value=CondSig_mesureTemp_Vsub
  Out1 : Outport  ConcatenationDimension=1
  wires:
  In1/1 -> Sum/1, Divide/1  "Ohms"
  Sum/1 -> Divide/2
  Constant/1 -> Sum/2
  Divide/1 -> Gain/1
  Vsub/1 -> Subtract/2
  Subtract/1 -> Gain1/1
  Gain1/1 -> Saturation/1
  Saturation/1 -> Out1/1
  Gain/1 -> Subtract/1  "V (3.10-1.95)"

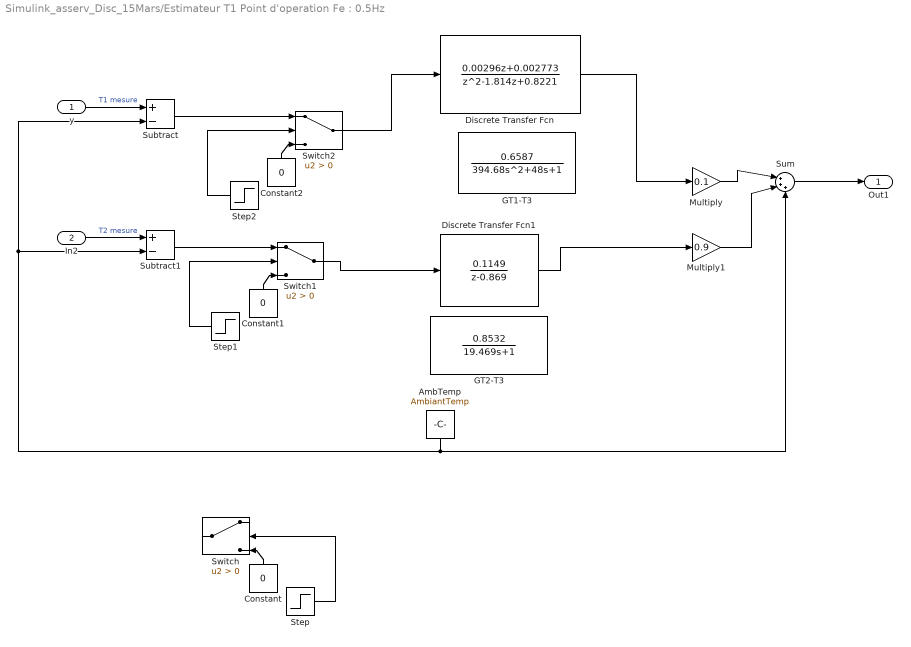
== system Simulink_asserv_Disc_15Mars/Estimateur T1 Point d'operation Fe : 0.5Hz ==
  y : Inport
  In2 : Inport  Port=2
  AmbTemp : Constant  Value=AmbiantTemp  SampleTime=2
  Constant : Constant  Value=0
  Constant1 : Constant  Value=0  SampleTime=2
  Constant2 : Constant  Value=0  SampleTime=2
  Discrete Transfer Fcn : DiscreteTransferFcn  Numerator=[0 0.00296 0.002773]  Denominator=[1 -1.814 0.8221]
  Discrete Transfer Fcn1 : DiscreteTransferFcn  Numerator=[0 0.1149]  Denominator=[1 -0.869]
  GT1-T3 : TransferFcn  Numerator=[0.6587]  Denominator=[394.68 48 1]
  GT2-T3 : TransferFcn  Numerator=[0.8532]  Denominator=[19.469 1]
  Multiply : Gain  Gain=0.1
  Multiply1 : Gain  Gain=0.9
  Step : Step  Time=setupDelay  SampleTime=0
  Step1 : Step  Time=setupDelay  SampleTime=periodeEchant
  Step2 : Step  Time=setupDelay  SampleTime=periodeEchant
  Subtract : Sum  Inputs=+-
  Subtract1 : Sum  Inputs=+-
  Sum : Sum  Inputs=|+++
  Switch : Switch  Criteria=u2 > Threshold  SaturateOnIntegerOverflow=off  InputSameDT=off
  Switch1 : Switch  Criteria=u2 > Threshold  SaturateOnIntegerOverflow=off  InputSameDT=off
  Switch2 : Switch  Criteria=u2 > Threshold  SaturateOnIntegerOverflow=off  InputSameDT=off
  Out1 : Outport  SampleTime=periodeEchant
  wires:
  In2/1 -> Subtract1/1  "T2 mesure"
  Multiply/1 -> Sum/1
  Multiply1/1 -> Sum/2
  y/1 -> Subtract/1  "T1 mesure"
  Sum/1 -> Out1/1
  Discrete Transfer Fcn/1 -> Multiply/1
  Discrete Transfer Fcn1/1 -> Multiply1/1
  AmbTemp/1 -> Subtract1/2, Subtract/2, Sum/3
  Constant1/1 -> Switch1/3
  Constant2/1 -> Switch2/3
  Step2/1 -> Switch2/2
  Subtract/1 -> Switch2/1
  Switch2/1 -> Discrete Transfer Fcn/1
  Constant/1 -> Switch/3
  Step/1 -> Switch/2
  Subtract1/1 -> Switch1/1
  Step1/1 -> Switch1/2
  Switch1/1 -> Discrete Transfer Fcn1/1

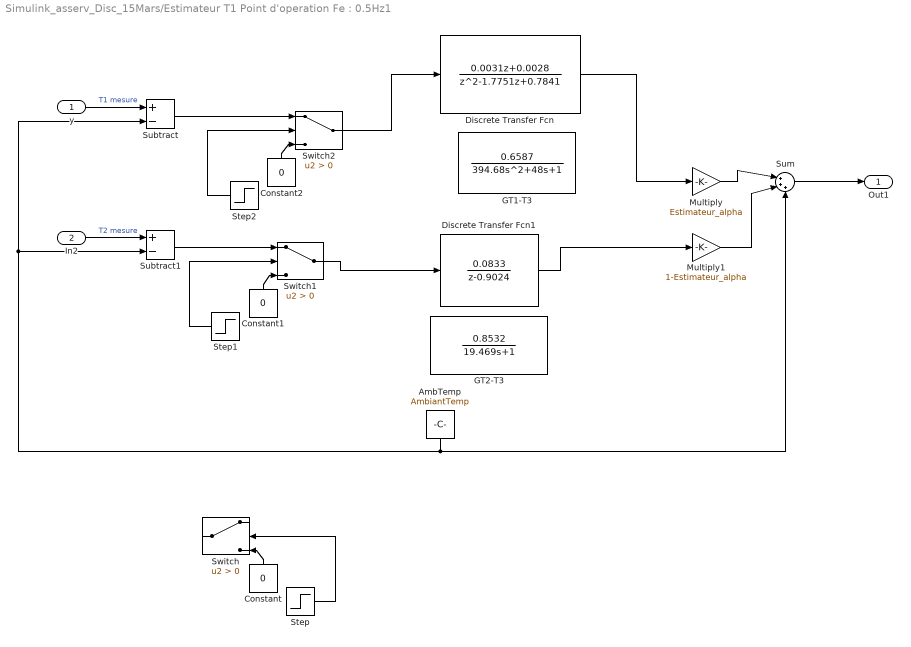
== system Simulink_asserv_Disc_15Mars/Estimateur T1 Point d'operation Fe : 0.5Hz1 ==
  y : Inport
  In2 : Inport  Port=2
  AmbTemp : Constant  Value=AmbiantTemp  SampleTime=2
  Constant : Constant  Value=0
  Constant1 : Constant  Value=0  SampleTime=2
  Constant2 : Constant  Value=0  SampleTime=2
  Discrete Transfer Fcn : DiscreteTransferFcn  Numerator=[0 0.0031 0.0028]  Denominator=[1 -1.7751 0.7841]
  Discrete Transfer Fcn1 : DiscreteTransferFcn  Numerator=[0 0.0833]  Denominator=[1 -0.9024]
  GT1-T3 : TransferFcn  Numerator=[0.6587]  Denominator=[394.68 48 1]
  GT2-T3 : TransferFcn  Numerator=[0.8532]  Denominator=[19.469 1]
  Multiply : Gain  Gain=Estimateur_alpha
  Multiply1 : Gain  Gain=1-Estimateur_alpha
  Step : Step  Time=setupDelay  SampleTime=0
  Step1 : Step  Time=setupDelay  SampleTime=periodeEchant
  Step2 : Step  Time=setupDelay  SampleTime=periodeEchant
  Subtract : Sum  Inputs=+-
  Subtract1 : Sum  Inputs=+-
  Sum : Sum  Inputs=|+++
  Switch : Switch  Criteria=u2 > Threshold  SaturateOnIntegerOverflow=off  InputSameDT=off
  Switch1 : Switch  Criteria=u2 > Threshold  SaturateOnIntegerOverflow=off  InputSameDT=off
  Switch2 : Switch  Criteria=u2 > Threshold  SaturateOnIntegerOverflow=off  InputSameDT=off
  Out1 : Outport  SampleTime=periodeEchant
  wires:
  In2/1 -> Subtract1/1  "T2 mesure"
  Multiply/1 -> Sum/1
  Multiply1/1 -> Sum/2
  y/1 -> Subtract/1  "T1 mesure"
  Sum/1 -> Out1/1
  Discrete Transfer Fcn/1 -> Multiply/1
  Discrete Transfer Fcn1/1 -> Multiply1/1
  AmbTemp/1 -> Subtract1/2, Subtract/2, Sum/3
  Constant1/1 -> Switch1/3
  Constant2/1 -> Switch2/3
  Step2/1 -> Switch2/2
  Subtract/1 -> Switch2/1
  Switch2/1 -> Discrete Transfer Fcn/1
  Constant/1 -> Switch/3
  Step/1 -> Switch/2
  Subtract1/1 -> Switch1/1
  Step1/1 -> Switch1/2
  Switch1/1 -> Discrete Transfer Fcn1/1

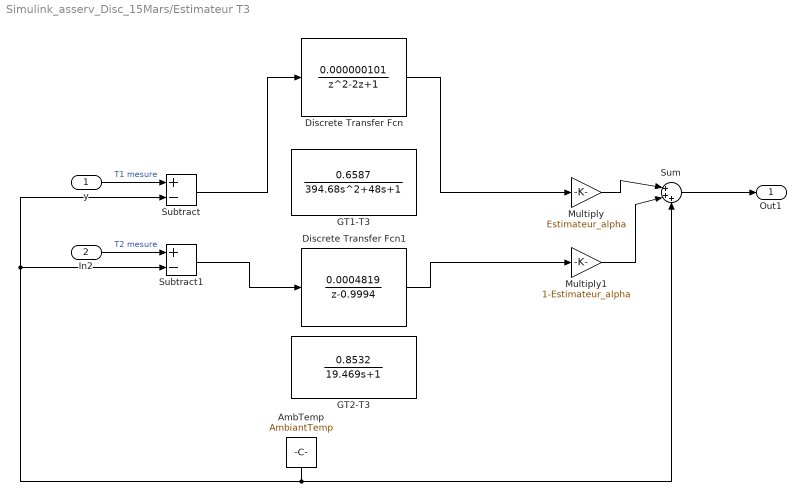
== system Simulink_asserv_Disc_15Mars/Estimateur T3 ==
  y : Inport
  In2 : Inport  Port=2
  AmbTemp : Constant  Value=AmbiantTemp
  Discrete Transfer Fcn : DiscreteTransferFcn  Numerator=[0.000000101]  Denominator=[1 -2 1]
  Discrete Transfer Fcn1 : DiscreteTransferFcn  Numerator=[0.0004819]  Denominator=[1 -0.9994]
  GT1-T3 : TransferFcn  Numerator=[0.6587]  Denominator=[394.68 48 1]
  GT2-T3 : TransferFcn  Numerator=[0.8532]  Denominator=[19.469 1]
  Multiply : Gain  Gain=Estimateur_alpha
  Multiply1 : Gain  Gain=1-Estimateur_alpha
  Subtract : Sum  Inputs=+-
  Subtract1 : Sum  Inputs=+-
  Sum : Sum  Inputs=|+++
  Out1 : Outport
  wires:
  In2/1 -> Subtract1/1  "T2 mesure"
  Multiply/1 -> Sum/1
  Multiply1/1 -> Sum/2
  y/1 -> Subtract/1  "T1 mesure"
  Subtract/1 -> Discrete Transfer Fcn/1
  Subtract1/1 -> Discrete Transfer Fcn1/1
  Sum/1 -> Out1/1
  AmbTemp/1 -> Sum/3, Subtract1/2, Subtract/2
  Discrete Transfer Fcn/1 -> Multiply/1
  Discrete Transfer Fcn1/1 -> Multiply1/1

== system Simulink_asserv_Disc_15Mars/Simulateur PWM Arduino1 ==
  In1 : Inport
  Gain1 : Gain  Gain=1/255
  Gain2 : Gain  Gain=5
  PWM : simulink/Discontinuities/PWM  DisableCoverage=on  Period=0.00204  InitialDelay=0  DisallowZeroDutyCycle=off  RunAtFixedTimeIntervals=off  SampleTime=0.1
  Out1 : Outport
  wires:
  Gain1/1 -> PWM/1
  PWM/1 -> Gain2/1
  In1/1 -> Gain1/1
  Gain2/1 -> Out1/1

== system Simulink_asserv_Disc_15Mars/Simulateur PWM Arduino2 ==
  In1 : Inport
  Gain1 : Gain  Gain=1/255
  Gain2 : Gain  Gain=5
  PWM : simulink/Discontinuities/PWM  DisableCoverage=on  Period=0.00204  InitialDelay=0  DisallowZeroDutyCycle=off  RunAtFixedTimeIntervals=off  SampleTime=0.1
  Out1 : Outport
  wires:
  Gain1/1 -> PWM/1
  PWM/1 -> Gain2/1
  In1/1 -> Gain1/1
  Gain2/1 -> Out1/1

== system Simulink_asserv_Disc_15Mars/Simulateur PWM Arduino3 ==
  In1 : Inport
  Gain1 : Gain  Gain=1/255
  Gain2 : Gain  Gain=5
  PWM : simulink/Discontinuities/PWM  DisableCoverage=on  Period=0.00204  InitialDelay=0  DisallowZeroDutyCycle=off  RunAtFixedTimeIntervals=off  SampleTime=0.1
  Out1 : Outport
  wires:
  Gain1/1 -> PWM/1
  PWM/1 -> Gain2/1
  In1/1 -> Gain1/1
  Gain2/1 -> Out1/1

== system Simulink_asserv_Disc_15Mars/ThermoResistance ==
  In1 : Inport  Partition=on  PartitionDimension=1  PartitionWidth=1  PartitionOffset=0
  A : Constant  Value=ThermoRes_SH_A
  B : Constant  Value=ThermoRes_SH_B
  C : Constant  Value=ThermoRes_SH_C
  D : Constant  Value=ThermoRes_SH_D
  For Each : ForEach  DisableCoverage=on
  MATLAB Function : MATLAB Function  TreatAsAtomicUnit=on
  R_nom : Constant  Value=ThermoRes_SH_R_nom
  y : Outport  ConcatenationDimension=1
  wires:
  In1/1 -> MATLAB Function/1(u)
  MATLAB Function/1(y) -> y/1
  A/1 -> MATLAB Function/2(A)
  B/1 -> MATLAB Function/3(B)
  C/1 -> MATLAB Function/4(C)
  D/1 -> MATLAB Function/5(D)
  R_nom/1 -> MATLAB Function/6(R_nom)

== system Simulink_asserv_Disc_15Mars/ThermoResistance1 ==
  In1 : Inport  Partition=on  PartitionDimension=1  PartitionWidth=1  PartitionOffset=0
  A : Constant  Value=ThermoRes_SH_A
  B : Constant  Value=ThermoRes_SH_B
  C : Constant  Value=ThermoRes_SH_C
  D : Constant  Value=ThermoRes_SH_D
  For Each : ForEach  DisableCoverage=on
  MATLAB Function : MATLAB Function  TreatAsAtomicUnit=on
  R_nom : Constant  Value=ThermoRes_SH_R_nom
  y : Outport  ConcatenationDimension=1
  wires:
  In1/1 -> MATLAB Function/1(u)
  MATLAB Function/1(y) -> y/1
  A/1 -> MATLAB Function/2(A)
  B/1 -> MATLAB Function/3(B)
  C/1 -> MATLAB Function/4(C)
  D/1 -> MATLAB Function/5(D)
  R_nom/1 -> MATLAB Function/6(R_nom)

== system Simulink_asserv_Disc_15Mars/ThermoResistance2 ==
  In1 : Inport  Partition=on  PartitionDimension=1  PartitionWidth=1  PartitionOffset=0
  A : Constant  Value=ThermoRes_SH_A
  B : Constant  Value=ThermoRes_SH_B
  C : Constant  Value=ThermoRes_SH_C
  D : Constant  Value=ThermoRes_SH_D
  For Each : ForEach  DisableCoverage=on
  MATLAB Function : MATLAB Function  TreatAsAtomicUnit=on
  R_nom : Constant  Value=ThermoRes_SH_R_nom
  y : Outport  ConcatenationDimension=1
  wires:
  In1/1 -> MATLAB Function/1(u)
  MATLAB Function/1(y) -> y/1
  A/1 -> MATLAB Function/2(A)
  B/1 -> MATLAB Function/3(B)
  C/1 -> MATLAB Function/4(C)
  D/1 -> MATLAB Function/5(D)
  R_nom/1 -> MATLAB Function/6(R_nom)

== system Simulink_asserv_Disc_15Mars/ThermoResistance3 ==
  In1 : Inport  Partition=on  PartitionDimension=1  PartitionWidth=1  PartitionOffset=0
  A : Constant  Value=ThermoRes_SH_A
  B : Constant  Value=ThermoRes_SH_B
  C : Constant  Value=ThermoRes_SH_C
  D : Constant  Value=ThermoRes_SH_D
  For Each : ForEach  DisableCoverage=on
  MATLAB Function : MATLAB Function  TreatAsAtomicUnit=on
  R_nom : Constant  Value=ThermoRes_SH_R_nom
  y : Outport  ConcatenationDimension=1
  wires:
  In1/1 -> MATLAB Function/1(u)
  MATLAB Function/1(y) -> y/1
  A/1 -> MATLAB Function/2(A)
  B/1 -> MATLAB Function/3(B)
  C/1 -> MATLAB Function/4(C)
  D/1 -> MATLAB Function/5(D)
  R_nom/1 -> MATLAB Function/6(R_nom)

== system Simulink_asserv_Disc_15Mars/ThermoResistance_ ==
  In1 : Inport  Partition=on  PartitionDimension=1  PartitionWidth=1  PartitionOffset=0
  A : Constant  Value=ThermoRes_SH_A
  B : Constant  Value=ThermoRes_SH_B
  C : Constant  Value=ThermoRes_SH_C
  D : Constant  Value=ThermoRes_SH_D
  For Each : ForEach  DisableCoverage=on
  MATLAB Function : MATLAB Function  TreatAsAtomicUnit=on
  R_nom : Constant  Value=ThermoRes_SH_R_nom
  Out1 : Outport  ConcatenationDimension=1
  wires:
  A/1 -> MATLAB Function/2(A)
  D/1 -> MATLAB Function/5(D)
  B/1 -> MATLAB Function/3(B)
  R_nom/1 -> MATLAB Function/6(R_nom)
  C/1 -> MATLAB Function/4(C)
  MATLAB Function/1(y) -> Out1/1
  In1/1 -> MATLAB Function/1(u)

== matlab function Simulink_asserv_Disc_15Mars/Calculs Arduinos3/MATLAB Function1 ==
  data: u input; y output; A input; B input; C input; D input; Rnom input
function y = fcn(u, A, B, C, D, Rnom)
    invT = A + B*log(u/Rnom) + C*(log(u/Rnom))^2 + D*(log(u/Rnom))^3;
    T = (1/invT) - 273.15;
y = T;

== matlab function Simulink_asserv_Disc_15Mars/Calculs Arduinos1/MATLAB Function ==
  data: u input; y output; Vref input; Rpull input
function y = fcn(u, Vref, Rpull)

y = Rpull * (u/(Vref-u));

== matlab function Simulink_asserv_Disc_15Mars/ThermoResistance2/MATLAB Function ==
  data: u input; y output; A input; B input; C input; D input; R_nom input
function y = fcn(u, A, B, C, D, R_nom)
   
y = R_nom * exp(A + (B/(u+273.15)) + (C/((u + 273.15)^2)) + (D/((u + 273.15)^3)));

== matlab function Simulink_asserv_Disc_15Mars/ThermoResistance3/MATLAB Function ==
  data: u input; y output; A input; B input; C input; D input; R_nom input
function y = fcn(u, A, B, C, D, R_nom)
   
y = R_nom * exp(A + (B/(u+273.15)) + (C/((u + 273.15)^2)) + (D/((u + 273.15)^3)));

== matlab function Simulink_asserv_Disc_15Mars/Calculs Arduinos4/MATLAB Function ==
  data: u input; y output; Vref input; Rpull input
function y = fcn(u, Vref, Rpull)

y = Rpull * (u/(Vref-u));

== matlab function Simulink_asserv_Disc_15Mars/Calculs Arduinos4/MATLAB Function1 ==
  data: u input; y output; A input; B input; C input; D input; Rnom input
function y = fcn(u, A, B, C, D, Rnom)
    invT = A + B*log(u/Rnom) + C*(log(u/Rnom))^2 + D*(log(u/Rnom))^3;
    T = (1/invT) - 273.15;
y = T;

== matlab function Simulink_asserv_Disc_15Mars/ThermoResistance_/MATLAB Function ==
  data: u input; y output; A input; B input; C input; D input; R_nom input
function y = fcn(u, A, B, C, D, R_nom)
   
y = R_nom * exp(A + (B/(u+273.15)) + (C/((u + 273.15)^2)) + (D/((u + 273.15)^3)));

== matlab function Simulink_asserv_Disc_15Mars/ThermoResistance/MATLAB Function ==
  data: u input; y output; A input; B input; C input; D input; R_nom input
function y = fcn(u, A, B, C, D, R_nom)
   
y = R_nom * exp(A + (B/(u+273.15)) + (C/((u + 273.15)^2)) + (D/((u + 273.15)^3)));

== matlab function Simulink_asserv_Disc_15Mars/Calculs Arduinos/MATLAB Function ==
  data: u input; y output; Vref input; Rpull input
function y = fcn(u, Vref, Rpull)

y = Rpull * (u/(Vref-u));

== matlab function Simulink_asserv_Disc_15Mars/Calculs Arduinos/MATLAB Function1 ==
  data: u input; y output; A input; B input; C input; D input; Rnom input
function y = fcn(u, A, B, C, D, Rnom)
    invT = A + B*log(u/Rnom) + C*(log(u/Rnom))^2 + D*(log(u/Rnom))^3;
    T = (1/invT) - 273.15;
y = T;

== matlab function Simulink_asserv_Disc_15Mars/Calculs Arduinos1/MATLAB Function1 ==
  data: u input; y output; A input; B input; C input; D input; Rnom input
function y = fcn(u, A, B, C, D, Rnom)
    invT = A + B*log(u/Rnom) + C*(log(u/Rnom))^2 + D*(log(u/Rnom))^3;
    T = (1/invT) - 273.15;
y = T;

== matlab function Simulink_asserv_Disc_15Mars/ThermoResistance1/MATLAB Function ==
  data: u input; y output; A input; B input; C input; D input; R_nom input
function y = fcn(u, A, B, C, D, R_nom)
   
y = R_nom * exp(A + (B/(u+273.15)) + (C/((u + 273.15)^2)) + (D/((u + 273.15)^3)));

== matlab function Simulink_asserv_Disc_15Mars/Calculs Arduinos2/MATLAB Function ==
  data: u input; y output; Vref input; Rpull input
function y = fcn(u, Vref, Rpull)

y = Rpull * (u/(Vref-u));

== matlab function Simulink_asserv_Disc_15Mars/Calculs Arduinos2/MATLAB Function1 ==
  data: u input; y output; A input; B input; C input; D input; Rnom input
function y = fcn(u, A, B, C, D, Rnom)
    invT = A + B*log(u/Rnom) + C*(log(u/Rnom))^2 + D*(log(u/Rnom))^3;
    T = (1/invT) - 273.15;
y = T;

== matlab function Simulink_asserv_Disc_15Mars/Calculs Arduinos3/MATLAB Function ==
  data: u input; y output; Vref input; Rpull input
function y = fcn(u, Vref, Rpull)

y = Rpull * (u/(Vref-u));
